simulink model "Case2_CLF_CBF_QP_Controller"  (R2026a)
settings: Solver=VariableStepAuto  StopTime=30
PreLoadFcn:
  | % Define variants
  | VSS_PATH_CTRL_PURE_PURSUIT=Simulink.Variant('VSS_PATH_CTRL_MODE==1');
  | VSS_PATH_CTRL_REAR_WHEEL=Simulink.Variant('VSS_PATH_CTRL_MODE==2');
  | % Select default variant
  | VSS_PATH_CTRL_MODE =1;
  | 
  | 
  | % Longitudinal PID
  | LongitudinalPID.Kp = 20;
  | LongitudinalPID.Ki = 0;
  | LongitudinalPID.Kd = 0;
  | LongitudinalPID.N = 100;
  | LongitudinalPID.MaxAccel = 80;
  | LongitudinalPID.SampleTime = 0.01;
  | 
  | % Steering PID
  | SteeringPID.Kp = 60;
  | SteeringPID.Ki = 0;
  | SteeringPID.Kd = 5;
  | SteeringPID.N = 10;
  | SteeringPID.MaxSpeed =  10;
  | SteeringPID.MinSpeed = -10;
  | SteeringPID.SampleTime = 0.01;
  | 
  | 
  | 
  | setSMVehicleVisuParameters;
  | 
  | % Load planner commands
  | load('PlannerCmdTests.mat');
  | % Assign one for testing:
  | plannerCmd = plannerCmdFwd;
  | % plannerCmd  = plannerCmdFwdBwd;
  | 
  | % Bus structure definition
  | load('PlannerBusStruct.mat');
  | 
  | % Rear Wheel Controller Parameters
  | RW.k_e = 0.2;    % 0.1
  | RW.k_theta = 1;   % 0.75
  | RW.SampleTime =  0.1;
  | RW.GoalRadius = 0.3;
  | 
  | % Pure pursuit parameters
  | PP.DesiredLinearVel = 5;
  | PP.MaxAngularVel  = 10;
  | PP.LookaheadDist  = 1;
  | PP.Wheelbase = 4;
  | PP.GoalRadius = 0.1;
  | PP.SampleTime = 0.1;
  | PP.LongitudinalPID.Kp = 20;
  | PP.LongitudinalPID.Ki = 0;
  | PP.LongitudinalPID.Kd = 0;
  | PP.LongitudinalPID.N = 100;
  | PP.LongitudinalPID.MaxLongAccel =  80;
  | PP.LongitudinalPID.MinLongAccel = -80;
  | 
  | % Spline ref
  | splineRef = [ 0 0 0;[plannerCmd.PathMatrix(1:plannerCmd.PathLengths(1),1:2,1),0*ones(length(plannerCmd.PathMatrix(1:plannerCmd.PathLengths(1),1,1)),1)]];
values from neighbouring files (symbols this model uses):
  m = max(2, ceil(Lseg/ds))    [Trajectory.m]    (also in plot_nmpc_result.m = NaN)
  s = [0; cumsum(hypot(diff(xs),diff(ys)))]    [Trajectory.m]    (also in plot_parking_mpc.m = evalin('base',name); plot_result.m = out.(names{k}))
  trajMatrix = [tvec, xd, yd, thd, vd, wd]    [Trajectory.m]    (also in plot_parking_mpc.m = evalin('base','trajMatrix'); plot_result.m = evalin('base','trajMatrix'))
undefined symbols (not defined in the file or in its folder): DiscIntNeverNeededParam, smvv, X, Y, Z
libraries: sm_lib x527, sm_vehicle_slalom_lib x48, fl_lib x40, fl_ps_legacy_lib x28, nesl_utility x13
(part 1 of 15)
settings Model: Creator=csantacr  LastModifiedBy=Sea
settings DataIOCC: LoggingToFile=on
settings SimscapeCC: SimscapeNormalizeSystem=off  SimscapeNominalValues="[{\"value\":\"1\",\"unit\":\"A\"},{\"value\":\"1\",\"unit\":\"bar\"},{\"value\":\"1\",\"unit\":\"cm^2\"},{\"value\":\"1\",\"unit\":\"cm^3/s\"},{\"value\":\"1\",\"unit\":\"kJ/kg\"},{\"value\":\"1\",\"unit\":\"kW\"},{\"value\":\"1\",\"unit\":\"l\"},{\"value\":\"1\",\"unit\":\"N\"},{\"value\":\"1\",\"unit\":\"N*m\"},{\"value\":\"1\",\"unit\":\"V\"}]"  SimscapeLogType=none  SimscapeLogDataHistory=5000.0
settings ExplorerConfigSet: InternalSimMechanicsExplorerSettings="<ExplorerConfiguration><canonicalview>default</canonicalview><AnimationSetting><BasePlaybackSpeed>1.0</BasePlaybackSpeed><PlaybackSpeedFactor>1.0</PlaybackSpeedFactor></AnimationSetting><TilePanel><TileInfo><Tiles Columns=\"1\" Count=\"2\" Rows=\"2\"><Column Weight=\"1\"/><Row Weight=\"0.4993\"/><Row Weight=\"0.5007\"/><Tile Height=\"1\" Width=\"1\" X=\"0\" Y=\"0\"/><Tile Height=\"1\" Width=\"1\" X=\"0\" Y=\"1\"/></Tiles></TileInfo><SceneInfo><SceneViewer><BGColor><R>0.60000002384185791</R><G>0.60000002384185791</G><B>0.60000002384185791</B></BGColor><Camera><DoPerspective>off</DoPerspective><Position><X>122.753178902162432</X><Y>-60.2531801004264622</Y><Z>85.3731797239170476</Z></Position><Center><X>37.3783324220490201</X><Y>25.1216663796874506</Y><Z>-0.00166675619682621345</Z></Center><Up><X>-0.408248290463863073</X><Y>0.408248290463863073</Y><Z>0.816496580927726145</Z></Up><ViewLimDist>1</ViewLimDist><YLim>29.4844991357607569</YLim><XLim>45.8841613769531307</XLim></Camera></SceneViewer><SceneViewer><BGColor><R>0.60000002384185791</R><G>0.60000002384185791</G><B>0.60000002384185791</B></BGColor><Camera><DoPerspective>on</DoPerspective><Position><X>8</X><Y>0</Y><Z>2</Z></Position><Center><X>0</X><Y>0.25</Y><Z>1.30299999999999994</Z></Center><Up><X>-2.22044604925031308e-16</X><Y>0</Y><Z>1</Z></Up><ViewLimDist>1</ViewLimDist><YLim>0.466307658154998583</YLim><XLim>0.72353341648828684</XLim></Camera></SceneViewer></SceneInfo></TilePanel><MechEditorPanel><Cameras><Camera><Id>Camera1</Id><Value><Name>DriverCamera</Name><NativeCamera><PositionTrackingFeature>Robot_Bicycle_Model.Visualizer.SM_Car_Visu.Vehicle1.Drivers_View_Cam.F</PositionTrackingFeature><CenterTrackingFeature>Robot_Bicycle_Model.Visualizer.SM_Car_Visu.Vehicle1.Drivers_View_Cam.F</CenterTrackingFeature><UpVectorTrackingFeature>Robot_Bicycle_Model.Visualizer.SM_Car_Visu.Vehicle1.Drivers_View_Cam.F</UpVectorTrackingFeature><CenterTrackingOrigin>off</CenterTrackingOrigin><CenterTrackingDirection>+X</CenterTrackingDirection><UpVectorTrackingDirection>+Z</UpVectorTrackingDirection></NativeCamera></Value></Camera><Camera><Id>Camera2</Id><Value><Name>FollowerX</Name><NativeCamera><PositionTrackingFeature>Robot_Bicycle_Model.Visualizer.SM_Car_Visu.Cameras_Frames.Front_View_Cam.F</PositionTrackingFeature><CenterTrackingFeature>Robot_Bicycle_Model.Visualizer.SM_Car_Visu.Vehicle1.Drivers_View_Cam.F</CenterTrackingFeature><UpVectorTrackingFeature>Robot_Bicycle_Model.Visualizer.SM_Car_Visu.Cameras_Frames.Front_View_Cam.F</UpVectorTrackingFeature><CenterTrackingOrigin>on</CenterTrackingOrigin><UpVectorTrackingDirection>-X</UpVectorTrackingDirection></NativeCamera></Value></Camera></Cameras><GfxPanelCameraMap><MapElement CameraMLId=\"Camera2\" GfxPanelIndex=\"1\"/></GfxPanelCameraMap><VideoCreator><PlaybackSpeedRatio>1.0</PlaybackSpeedRatio><FrameRate>30</FrameRate><VideoFormat>Motion JPEG AVI</VideoFormat><FrameSize>auto</FrameSize></VideoCreator></MechEditorPanel></ExplorerConfiguration>"

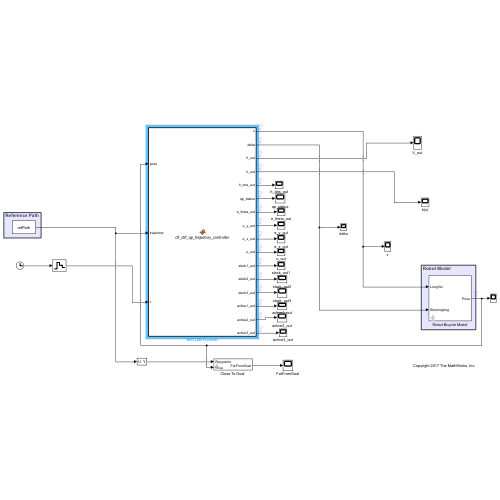
[thumbnail: Simulink's stored preview of the top-level diagram]
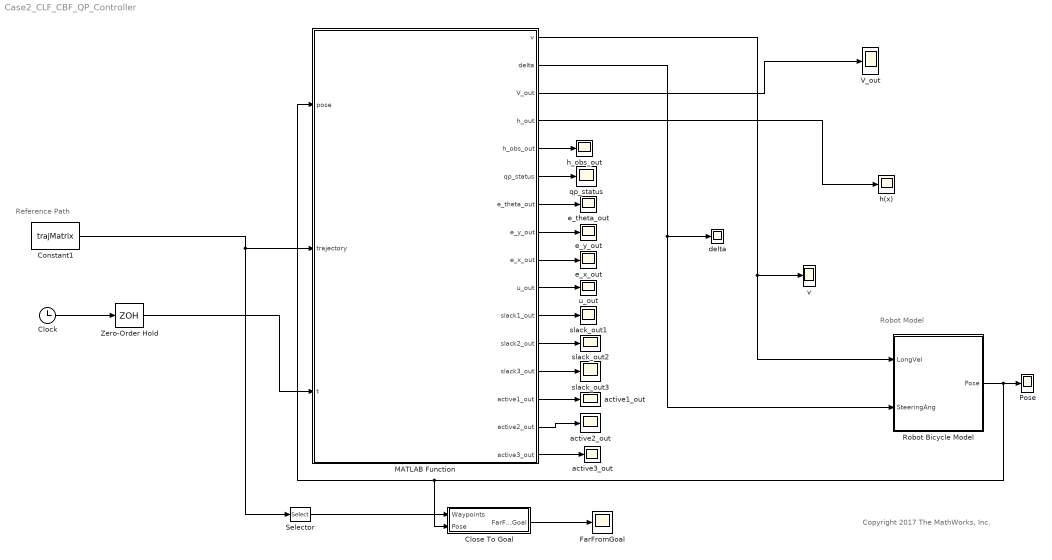
== system Case2_CLF_CBF_QP_Controller ==
  note: Copyright 2017 The MathWorks, Inc.
  note: Robot Model
  note: Reference Path
  Clock : Clock
  "Close To Goal " : Subsystem  mask{goalRadius=PP.GoalRadius}
      mask prompts: goalRadius "Goal Radius"
      mask DialogControl DescGroupVar Prompt: Close To Goal
      mask DialogControl DescTextVar Prompt: Check if close to goal
  Constant1 : Constant  Value=trajMatrix  VectorParams1D=off
      mask Display: disp('refPath');
  FarFromGoal : Scope
      settings: ActiveDisplayYMinimum=0.9  ActiveDisplayYMaximum=1.1  DataLoggingVariableName=ScopeData10
  MATLAB Function : MATLAB Function  TreatAsAtomicUnit=on  SystemSampleTime=0.01
  Pose : Scope
      settings: ActiveDisplayYMinimum=-6.9296030916089348  ActiveDisplayYMaximum=59.429979148987471  DataLoggingVariableName=pose_log
  Robot Bicycle Model : Subsystem  mask{wheelBase=3, maxLinearVelocity=80, sampleTime=5e-3, maxSteeringAng=60*pi/180, state_0=[0 16.36 0]}
      mask prompts: wheelBase "Wheel Base [m]"; maxLinearVelocity "Maximum Linear Velocity [m/s]"; sampleTime "Sample Time [s]"; maxSteeringAng "Max Steering Ang [rad]"; state_0 "Initial Condition [x,y,theta]"
  Selector : Selector  NumberOfDimensions=2  InputPortWidth=3  IndexOptions=Select all,Index vector (dialog)  Indices=[1 3],[2 3]  OutputSizes=1,1
  V_out : Scope
      settings: ActiveDisplayYMinimum=-0.032645596625243516  ActiveDisplayYMaximum=0.2938103696271917  DataLoggingVariableName=Vout_log
  Zero-Order Hold : ZeroOrderHold  SampleTime=0.01
  active1_out : Scope
      settings: ActiveDisplayYMinimum=-0.12499999999999997  ActiveDisplayYMaximum=1.125  DataLoggingVariableName=active1_log
  active2_out : Scope
      settings: DataLoggingVariableName=active2_log
  active3_out : Scope
      settings: DataLoggingVariableName=active3_log
  delta : Scope
      settings: ActiveDisplayYMinimum=-1.0989870972877505  ActiveDisplayYMaximum=1.1230265089850515  DataLoggingVariableName=delta_log
  e_theta_out : Scope
      settings: ActiveDisplayYMinimum=-1  ActiveDisplayYMaximum=1  DataLoggingVariableName=eth_log
  e_x_out : Scope
      settings: ActiveDisplayYMinimum=-3.0596180061562785  ActiveDisplayYMaximum=3.0448929725725327  DataLoggingVariableName=ex_log
  e_y_out : Scope
      settings: ActiveDisplayYMinimum=-1  ActiveDisplayYMaximum=1  DataLoggingVariableName=ey_log
  h(x) : Scope
      settings: ActiveDisplayYMinimum=-0.22434897213807364  ActiveDisplayYMaximum=1.9287865372378259  DataLoggingVariableName=h_log
  h_obs_out : Scope
      settings: ActiveDisplayYMinimum=-212.92680425947211  ActiveDisplayYMaximum=1992.0909004482746  DataLoggingVariableName=hobs_log
  qp_status : Scope
      settings: ActiveDisplayYMinimum=-1  ActiveDisplayYMaximum=1  DataLoggingVariableName=qp_log
  slack_out1 : Scope
      settings: DataLoggingVariableName=slack1_log
  slack_out2 : Scope
      settings: DataLoggingVariableName=slack2_log
  slack_out3 : Scope
      settings: DataLoggingVariableName=slack3_log
  u_out : Scope
      settings: ActiveDisplayYMinimum=-1  ActiveDisplayYMaximum=1  DataLoggingVariableName=ScopeData9
  v : Scope
      settings: ActiveDisplayYMinimum=-2.1757249365262057  ActiveDisplayYMaximum=4.581524428735853  DataLoggingVariableName=v_log
  wires:
  MATLAB Function/3(V_out) -> V_out/1
  Clock/1 -> Zero-Order Hold/1
  Zero-Order Hold/1 -> MATLAB Function/3(t)
  MATLAB Function/5(h_obs_out) -> h_obs_out/1
  Constant1/1 -> Selector/1, MATLAB Function/2(trajectory)
  Robot Bicycle Model/1(Pose) -> "Close To Goal "/2(Pose), MATLAB Function/1(pose), Pose/1
  MATLAB Function/4(h_out) -> h(x)/1
  Selector/1 -> "Close To Goal "/1(Waypoints)
  "Close To Goal "/1(FarFromGoal) -> FarFromGoal/1
  MATLAB Function/1(v) -> Robot Bicycle Model/1(LongVel), v/1
  MATLAB Function/2(delta) -> Robot Bicycle Model/2(SteeringAng), delta/1
  MATLAB Function/6(qp_status) -> qp_status/1
  MATLAB Function/7(e_theta_out) -> e_theta_out/1
  MATLAB Function/8(e_y_out) -> e_y_out/1
  MATLAB Function/9(e_x_out) -> e_x_out/1
  MATLAB Function/10(u_out) -> u_out/1
  MATLAB Function/11(slack1_out) -> slack_out1/1
  MATLAB Function/12(slack2_out) -> slack_out2/1
  MATLAB Function/13(slack3_out) -> slack_out3/1
  MATLAB Function/14(active1_out) -> active1_out/1
  MATLAB Function/15(active2_out) -> active2_out/1
  MATLAB Function/16(active3_out) -> active3_out/1

== system Case2_CLF_CBF_QP_Controller/Close To Goal  ==
  Waypoints : Inport
  Pose : Inport  Port=2
  " Extract Goal" : MATLAB Function  TreatAsAtomicUnit=on
  Data Type Conversion : DataTypeConversion  OutDataTypeStr=double  SaturateOnIntegerOverflow=off  RndMeth=Floor
  Dot Product : DotProduct  OutDataTypeStr=Inherit: Inherit via internal rule
  GoalRadius : Constant  Value=goalRadius
  Logical Operator : Logic  Operator=NOT  AllPortsSameDT=off  OutDataTypeStr=boolean
  Relational Operator : RelationalOperator  Operator=<=  OutDataTypeStr=boolean  RndMeth=Simplest  InputSameDT=off
  Selector : Selector  InputPortWidth=3  IndexOptions=Index vector (dialog)  Indices=[1 2]  OutputSizes=1
  Sqrt : Sqrt
  Subtract : Sum  Inputs=+-
  FarFromGoal : Outport  VectorParamsAs1DForOutWhenUnconnected=off
  wires:
  GoalRadius/1 -> Relational Operator/2
  Sqrt/1 -> Relational Operator/1
  Pose/1 -> Selector/1
  " Extract Goal"/1(Goal) -> Subtract/2
  Selector/1 -> Subtract/1
  Dot Product/1 -> Sqrt/1
  Relational Operator/1 -> Logical Operator/1
  Subtract/1 -> Dot Product/1, Dot Product/2
  Waypoints/1 -> " Extract Goal"/1(Waypoints)
  Logical Operator/1 -> Data Type Conversion/1
  Data Type Conversion/1 -> FarFromGoal/1

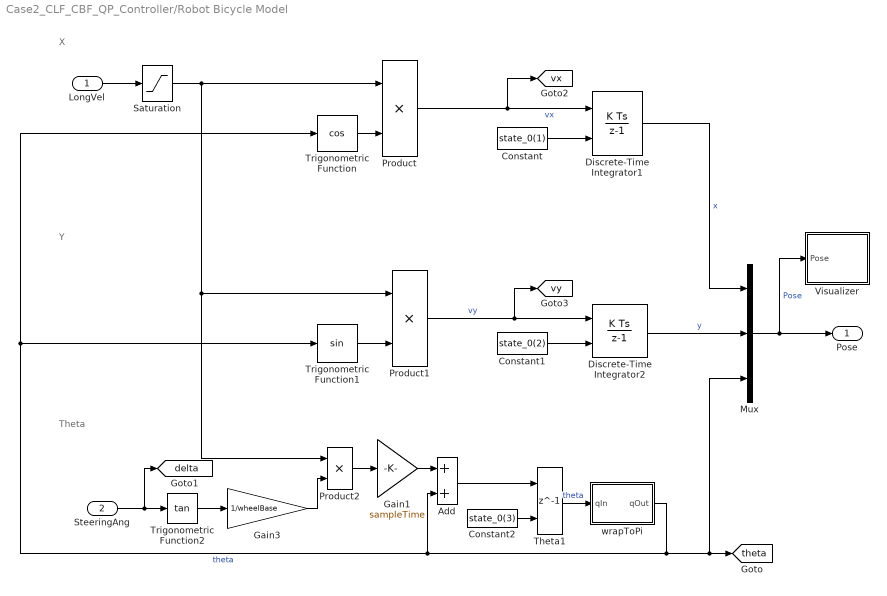
== system Case2_CLF_CBF_QP_Controller/Robot Bicycle Model ==
  note: X
  note: Y
  note: Theta
  LongVel : Inport
  SteeringAng : Inport  Port=2  SampleTime=sampleTime
  Add : Sum
  Constant : Constant  Value=state_0(1)
  Constant1 : Constant  Value=state_0(2)
  Constant2 : Constant  Value=state_0(3)
  Discrete-Time Integrator1 : DiscreteIntegrator  InitialConditionSource=external  SampleTime=-1  ICPrevOutput=DiscIntNeverNeededParam  ICPrevScaledInput=DiscIntNeverNeededParam
  Discrete-Time Integrator2 : DiscreteIntegrator  InitialConditionSource=external  SampleTime=-1  ICPrevOutput=DiscIntNeverNeededParam  ICPrevScaledInput=DiscIntNeverNeededParam
  Gain1 : Gain  Gain=sampleTime
  Gain3 : Gain  Gain=1/wheelBase
  Mux : Mux  Inputs=3
  Product : Product
  Product1 : Product
  Product2 : Product
  Saturation : Saturate  UpperLimit=maxLinearVelocity  LowerLimit=-maxLinearVelocity
  Theta1 : Delay  DelayLength=1  InitialConditionSource=Input port
      settings: InputPortMap=u0,p4
  Trigonometric Function : Trigonometry  Operator=cos
  Trigonometric Function1 : Trigonometry
  Trigonometric Function2 : Trigonometry  Operator=tan
  Visualizer : Subsystem
  wrapToPi : MATLAB Function  TreatAsAtomicUnit=on
      settings: CopyFcn=set_param(gcbh,'LinkStatus','none');
  Pose : Outport  VectorParamsAs1DForOutWhenUnconnected=off
  tag scope: delta=global, theta=global, vx=global, vy=global
  wires:
  wrapToPi/1(qOut) -> Trigonometric Function/1, Trigonometric Function1/1, Add/2, Mux/3, [theta]  "theta"
  Saturation/1 -> Product2/1, Product1/1, Product/1
  Mux/1 -> Pose/1, Visualizer/1(Pose)  "Pose"
  Theta1/1 -> wrapToPi/1(qIn)  "theta"
  Gain1/1 -> Add/1
  Add/1 -> Theta1/1
  Trigonometric Function/1 -> Product/2
  Product/1 -> [vx], Discrete-Time Integrator1/1  "vx"
  Trigonometric Function1/1 -> Product1/2
  Product1/1 -> [vy], Discrete-Time Integrator2/1  "vy"
  Product2/1 -> Gain1/1
  Constant2/1 -> Theta1/2
  Trigonometric Function2/1 -> Gain3/1
  Gain3/1 -> Product2/2
  Discrete-Time Integrator1/1 -> Mux/1  "x"
  Discrete-Time Integrator2/1 -> Mux/2  "y"
  Constant/1 -> Discrete-Time Integrator1/2
  Constant1/1 -> Discrete-Time Integrator2/2
  SteeringAng/1 -> [delta], Trigonometric Function2/1
  LongVel/1 -> Saturation/1

== system Case2_CLF_CBF_QP_Controller/Robot Bicycle Model/Visualizer ==
  Pose : Inport
  Demux : Demux  Outputs=3
  Demux1 : Demux  Outputs=2
  Earth_To_Body : Subsystem
  Extract_Vel_Steer : Subsystem
  Mux1 : Mux  Inputs=2
  Mux3 : Mux  Inputs=9
  SM_Car_Visu : Subsystem
  Terminator : Terminator
  wires:
  Demux/1 -> Mux3/1
  Demux/2 -> Mux3/2
  [theta] -> Mux3/3
  Pose/1 -> SM_Car_Visu/1(Pose_Rear), Demux/1
  Mux3/1 -> Extract_Vel_Steer/1(State)
  [vy] -> Mux1/2
  [vy] -> Mux3/5
  [vx] -> Mux3/4
  [delta] -> Mux3/7
  [vx] -> Mux1/1
  [thetaDot] -> Mux3/6
  Mux1/1 -> Earth_To_Body/1(w_v)
  [theta] -> Earth_To_Body/2(theta)
  Earth_To_Body/1(f_v) -> Demux1/1
  Demux1/1 -> Mux3/8
  Demux1/2 -> Mux3/9
  Extract_Vel_Steer/1(Long_Vel) -> SM_Car_Visu/2(Long_Vel)
  Extract_Vel_Steer/2(Steering_Ang) -> SM_Car_Visu/3(Steering_Angle)
  Demux/3 -> Terminator/1

== system Case2_CLF_CBF_QP_Controller/Robot Bicycle Model/Visualizer/Earth_To_Body ==
  w_v : Inport
  theta : Inport  Port=2
  Add : Sum
  Add1 : Sum
  Demux : Demux  Outputs=2
  Gain : Gain  Gain=-1
  Mux : Mux  Inputs=2
  Product{,1..3} (4 alike) : Product
  Trigonometric Function : Trigonometry
  Trigonometric Function1 : Trigonometry  Operator=cos
  f_v : Outport  VectorParamsAs1DForOutWhenUnconnected=off
  wires:
  Add1/1 -> Mux/2
  Product3/1 -> Add1/2
  Product2/1 -> Gain/1
  Trigonometric Function/1 -> Product1/1, Product2/2
  Add/1 -> Mux/1
  Mux/1 -> f_v/1
  Demux/2 -> Product3/2, Product1/2
  Product1/1 -> Add/2
  Product/1 -> Add/1
  Demux/1 -> Product2/1, Product/1
  w_v/1 -> Demux/1
  Trigonometric Function1/1 -> Product/2, Product3/1
  theta/1 -> Trigonometric Function/1, Trigonometric Function1/1
  Gain/1 -> Add1/1

== system Case2_CLF_CBF_QP_Controller/Robot Bicycle Model/Visualizer/Extract_Vel_Steer ==
  State : Inport
  Demux : Demux  Outputs=9
  Terminator{,1..6} (7 alike) : Terminator
  Long_Vel : Outport  VectorParamsAs1DForOutWhenUnconnected=off
  Steering_Ang : Outport  Port=2  VectorParamsAs1DForOutWhenUnconnected=off
  wires:
  State/1 -> Demux/1
  Demux/1 -> Terminator/1
  Demux/2 -> Terminator1/1
  Demux/3 -> Terminator2/1
  Demux/9 -> Terminator3/1
  Demux/4 -> Terminator4/1
  Demux/5 -> Terminator5/1
  Demux/6 -> Terminator6/1
  Demux/7 -> Steering_Ang/1
  Demux/8 -> Long_Vel/1

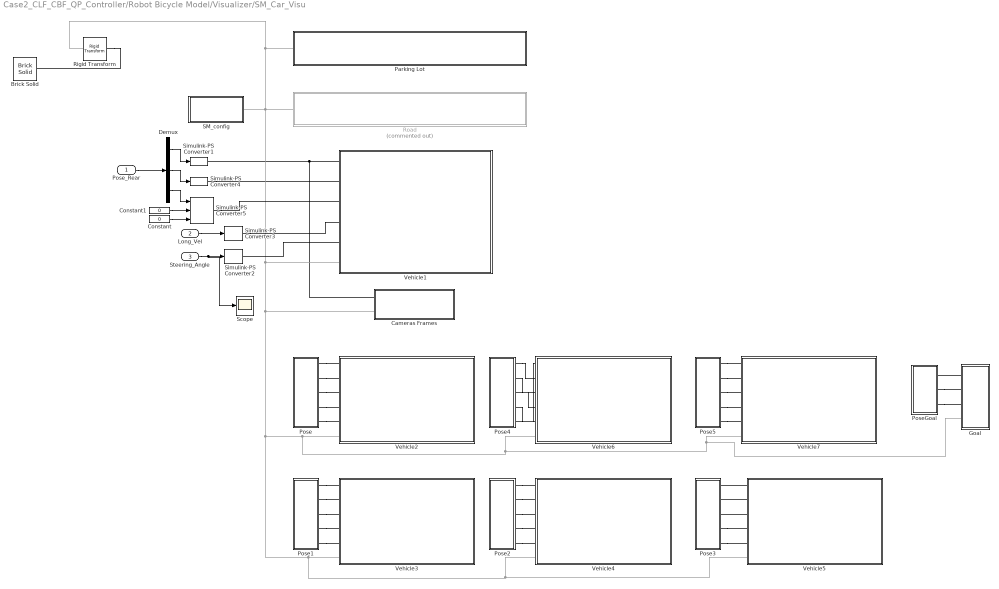
== system Case2_CLF_CBF_QP_Controller/Robot Bicycle Model/Visualizer/SM_Car_Visu ==
  Pose_Rear : Inport
  Long_Vel : Inport  Port=2
  Steering_Angle : Inport  Port=3
  Brick Solid : sm_lib/Body Elements/Brick Solid  BrickDimensions=[1 1 1]  BrickDimensionsUnits=m  ExportEntireGeometry=off  InertiaType=CalculateFromGeometry  BasedOnType=Density  Density=1000  DensityUnits=kg/m^3  Mass=1  MassUnits=kg  CenterOfMass=[0 0 0]  CenterOfMassUnits=m  MomentsOfInertia=[1 1 1]  MomentsOfInertiaUnits=kg*m^2  ProductsOfInertia=[0 0 0]  ProductsOfInertiaUnits=kg*m^2  GraphicType=FromGeometry  MarkerShape=Sphere  MarkerSize=10  GraphicVisPropType=SimpleVisualProperties  GraphicDiffuseColor=[0.3333 0.6667 0]  GraphicOpacity=1  GraphicSpecularColor=[0.5 0.5 0.5 1.0]  GraphicAmbientColor=[0.15 0.15 0.15 1.0]  GraphicEmissiveColor=[0.0 0.0 0.0 1.0]  GraphicShininess=75  DoExposeReferenceFrame=on  SerializedFrames=<Frames/>
  Cameras Frames : Subsystem
  Constant : Constant  Value=0
  Constant1 : Constant  Value=0
  Demux : Demux  Outputs=3
  Goal : Subsystem
  Parking Lot : Subsystem
  Pose : Subsystem
  Pose1 : Subsystem
  Pose2 : Subsystem
  Pose3 : Subsystem
  Pose4 : Subsystem
  Pose5 : Subsystem
  PoseGoal : Subsystem
  Rigid Transform : sm_lib/Frames and Transforms/Rigid Transform  RotationMethod=None  FollAlignAxisA=+X  BaseAlignAxisA=+Y  FollAlignAxisB=+Y  BaseAlignAxisB=+Z  RotationStandardAxis=+Z  RotationAngle=0  RotationAngleUnits=deg  RotationArbitraryAxis=[0 0 1]  RotationSequenceAxes=FollowerAxes  RotationSequence=XYX  RotationSequenceAngles=[0 0 0]  RotationSequenceAnglesUnits=deg  RotationMatrix=[1 0 0;0 1 0;0 0 1]  Quaternion=[1 0 0 0]  TranslationMethod=Cartesian  TranslationCartesianOffset=[0 17 0]  TranslationCartesianOffsetUnits=m  TranslationStandardAxis=+Z  TranslationStandardOffset=0  TranslationStandardOffsetUnits=m  TranslationROffset=0  TranslationROffsetUnits=m  TranslationThetaOffset=0  TranslationThetaOffsetUnits=deg  TranslationZOffset=0  TranslationZOffsetUnits=m
  Road : Subsystem  Commented=on
      mask Display: image(imread(fullfile(matlabroot,'toolbox','physmod','sm','smdemos','vehicle_slalom','images','sm_vehicle_slalom_road.png')));
  SM_config : Subsystem
  Scope : Scope
      settings: ActiveDisplayYMinimum=-1.10804  ActiveDisplayYMaximum=1.68533
  Simulink-PS Converter{1..4} (4 alike) : nesl_utility/Simulink-PS Converter  PhysicalDomain=network_engine_domain  SubClassName=ps_input  LeftPortType=input  RightPortType=output  PseudoPeriodic=off  Frequencies=[]  NoiseDistribution=none  NoiseParameters=[]  Unit=1  AffineConversion=off  FilteringAndDerivatives=filter  SimscapeFilterOrder=2  InputFilterTimeConstant=smvv.filter.t_c  UdotUserProvided=2
  Simulink-PS Converter5 : nesl_utility/Simulink-PS Converter  PhysicalDomain=network_engine_domain  SubClassName=ps_input  LeftPortType=input  RightPortType=output  PseudoPeriodic=off  Frequencies=[]  NoiseDistribution=none  NoiseParameters=[]  Unit=rad  AffineConversion=off  FilteringAndDerivatives=provide  SimscapeFilterOrder=2  InputFilterTimeConstant=smvv.filter.t_c  UdotUserProvided=2
  Vehicle1 : Subsystem
      mask Display: image(imread(fullfile(matlabroot,'toolbox','physmod','sm','smdemos','vehicle_slalom','images','sm_vehicle_slalom_vehicle.png')));
  Vehicle2 : Subsystem
      mask Display: image(imread(fullfile(matlabroot,'toolbox','physmod','sm','smdemos','vehicle_slalom','images','sm_vehicle_slalom_vehicle.png')));
  Vehicle3 : Subsystem
      mask Display: image(imread(fullfile(matlabroot,'toolbox','physmod','sm','smdemos','vehicle_slalom','images','sm_vehicle_slalom_vehicle.png')));
  Vehicle4 : Subsystem
      mask Display: image(imread(fullfile(matlabroot,'toolbox','physmod','sm','smdemos','vehicle_slalom','images','sm_vehicle_slalom_vehicle.png')));
  Vehicle5 : Subsystem
      mask Display: image(imread(fullfile(matlabroot,'toolbox','physmod','sm','smdemos','vehicle_slalom','images','sm_vehicle_slalom_vehicle.png')));
  Vehicle6 : Subsystem
      mask Display: image(imread(fullfile(matlabroot,'toolbox','physmod','sm','smdemos','vehicle_slalom','images','sm_vehicle_slalom_vehicle.png')));
  Vehicle7 : Subsystem
      mask Display: image(imread(fullfile(matlabroot,'toolbox','physmod','sm','smdemos','vehicle_slalom','images','sm_vehicle_slalom_vehicle.png')));
  wires:
  Demux/2 -> Simulink-PS Converter4/1
  Pose_Rear/1 -> Demux/1
  Demux/3 -> Simulink-PS Converter5/1
  Demux/1 -> Simulink-PS Converter1/1
  Steering_Angle/1 -> Scope/1, Simulink-PS Converter2/1
  Long_Vel/1 -> Simulink-PS Converter3/1
  Constant/1 -> Simulink-PS Converter5/3
  Constant1/1 -> Simulink-PS Converter5/2
  connections:
  Simulink-PS Converter4/RConn1 -- Vehicle1/LConn2
  Cameras Frames/LConn1 -- Vehicle1/LConn1 -- Simulink-PS Converter1/RConn1
  Road/LConn1 -- Parking Lot/LConn1 -- Rigid Transform/LConn1 -- SM_config/RConn1 -- Vehicle1/LConn6 -- Goal/LConn4 -- Vehicle7/LConn6 -- Vehicle6/LConn6 -- Vehicle2/LConn6 -- Vehicle5/LConn6 -- Vehicle4/LConn6 -- Vehicle3/LConn6 -- Cameras Frames/LConn2
  Vehicle1/LConn5 -- Simulink-PS Converter2/RConn1
  Simulink-PS Converter5/RConn1 -- Vehicle1/LConn3
  Simulink-PS Converter3/RConn1 -- Vehicle1/LConn4
  Pose/RConn1 -- Vehicle2/LConn1
  Pose/RConn2 -- Vehicle2/LConn2
  Pose/RConn3 -- Vehicle2/LConn3
  Pose/RConn4 -- Vehicle2/LConn4
  Pose/RConn5 -- Vehicle2/LConn5
  Pose1/RConn1 -- Vehicle3/LConn1
  Pose1/RConn2 -- Vehicle3/LConn2
  Pose1/RConn3 -- Vehicle3/LConn3
  Pose1/RConn4 -- Vehicle3/LConn4
  Pose1/RConn5 -- Vehicle3/LConn5
  Pose2/RConn1 -- Vehicle4/LConn1
  Pose2/RConn2 -- Vehicle4/LConn2
  Pose2/RConn3 -- Vehicle4/LConn3
  Pose2/RConn4 -- Vehicle4/LConn4
  Pose2/RConn5 -- Vehicle4/LConn5
  Vehicle5/LConn3 -- Pose3/RConn3
  Vehicle5/LConn2 -- Pose3/RConn2
  Vehicle5/LConn1 -- Pose3/RConn1
  Pose3/RConn4 -- Vehicle5/LConn4
  Pose3/RConn5 -- Vehicle5/LConn5
  Pose4/RConn3 -- Vehicle6/LConn4
  Pose4/RConn2 -- Vehicle6/LConn3
  Pose4/RConn1 -- Vehicle6/LConn2
  Pose4/RConn5 -- Vehicle6/LConn1
  Pose4/RConn4 -- Vehicle6/LConn5
  Pose5/RConn2 -- Vehicle7/LConn2
  Pose5/RConn1 -- Vehicle7/LConn1
  Pose5/RConn3 -- Vehicle7/LConn3
  Pose5/RConn4 -- Vehicle7/LConn4
  Pose5/RConn5 -- Vehicle7/LConn5
  Goal/LConn1 -- PoseGoal/RConn1
  PoseGoal/RConn2 -- Goal/LConn2
  PoseGoal/RConn3 -- Goal/LConn3
  Rigid Transform/RConn1 -- Brick Solid/RConn1

== system Case2_CLF_CBF_QP_Controller/Robot Bicycle Model/Visualizer/SM_Car_Visu/Cameras Frames ==
  Alignment xForm : sm_lib/Frames and Transforms/Rigid Transform  RotationMethod=AlignedAxes  FollAlignAxisA=+Z  BaseAlignAxisA=+X  FollAlignAxisB=+Y  BaseAlignAxisB=+Y  RotationStandardAxis=+Z  RotationAngle=0.0  RotationAngleUnits=deg  RotationArbitraryAxis=[0 0 1]  RotationSequenceAxes=FollowerAxes  RotationSequence=XYX  RotationSequenceAngles=[0 0 0]  RotationSequenceAnglesUnits=deg  RotationMatrix=[1 0 0; 0 1 0; 0 0 1]  Quaternion=[1 0 0 0]  TranslationMethod=None  TranslationCartesianOffset=[0 0 0]  TranslationCartesianOffsetUnits=m  TranslationStandardAxis=+Z  TranslationStandardOffset=0  TranslationStandardOffsetUnits=m  TranslationROffset=0  TranslationROffsetUnits=m  TranslationThetaOffset=0  TranslationThetaOffsetUnits=deg  TranslationZOffset=0  TranslationZOffsetUnits=m
  Front View xForm : sm_lib/Frames and Transforms/Rigid Transform  RotationMethod=None  FollAlignAxisA=+X  BaseAlignAxisA=+Y  FollAlignAxisB=+Y  BaseAlignAxisB=+Z  RotationStandardAxis=+Z  RotationAngle=0.0  RotationAngleUnits=deg  RotationArbitraryAxis=[0 0 1]  RotationSequenceAxes=FollowerAxes  RotationSequence=XYX  RotationSequenceAngles=[0 0 0]  RotationSequenceAnglesUnits=deg  RotationMatrix=[1 0 0; 0 1 0; 0 0 1]  Quaternion=[1 0 0 0]  TranslationMethod=Cartesian  TranslationCartesianOffset=smvv.cameras.frontView_offset  TranslationCartesianOffsetUnits=m  TranslationStandardAxis=+Z  TranslationStandardOffset=0  TranslationStandardOffsetUnits=m  TranslationROffset=0  TranslationROffsetUnits=m  TranslationThetaOffset=0  TranslationThetaOffsetUnits=deg  TranslationZOffset=0  TranslationZOffsetUnits=m
  Front View Cam : Subsystem
  Prismatic Joint : sm_lib/Joints/Prismatic Joint  JointMode=Normal  CompositeWrenchDir=FollowerOnBase  CompositeWrenchFrame=BaseFrame  SenseConstraintForce=off  SenseConstraintTorque=off  SenseTotalForce=off  SenseTotalTorque=off  PositionTargetSpecify=on  PositionTargetPriority=High  PositionTargetValue=smvv.vehicle.posX_0  PositionTargetValueUnits=m  VelocityTargetSpecify=off  VelocityTargetPriority=High  VelocityTargetValue=0  VelocityTargetValueUnits=m/s  EquilibriumPosition=0  EquilibriumPositionUnits=m  SpringStiffness=0  SpringStiffnessUnits=N/m  DampingCoefficient=0  DampingCoefficientUnits=N/(m/s)  LowerLimitSpecify=off  LowerLimitBound=-1  LowerLimitBoundUnits=m  LowerLimitStiffness=1e6  LowerLimitStiffnessUnits=N/m  LowerLimitDamping=1e3  LowerLimitDampingUnits=N/(m/s)  LowerLimitTransitionRegionWidth=1e-4  LowerLimitTransitionRegionWidthUnits=m  UpperLimitSpecify=off  UpperLimitBound=1  UpperLimitBoundUnits=m  UpperLimitStiffness=1e6  UpperLimitStiffnessUnits=N/m  UpperLimitDamping=1e3  UpperLimitDampingUnits=N/(m/s)  UpperLimitTransitionRegionWidth=1e-4  UpperLimitTransitionRegionWidthUnits=m  TorqueActuationMode=ComputedTorque  MotionActuationMode=InputMotion  SensePosition=off  SenseVelocity=off  SenseAcceleration=off  SenseTorqueForce=off  SenseLowerLimitTorqueForce=off  SenseUpperLimitTorqueForce=off
  Side View xForm : sm_lib/Frames and Transforms/Rigid Transform  RotationMethod=None  FollAlignAxisA=+X  BaseAlignAxisA=+Y  FollAlignAxisB=+Y  BaseAlignAxisB=+Z  RotationStandardAxis=+Z  RotationAngle=0.0  RotationAngleUnits=deg  RotationArbitraryAxis=[0 0 1]  RotationSequenceAxes=FollowerAxes  RotationSequence=XYX  RotationSequenceAngles=[0 0 0]  RotationSequenceAnglesUnits=deg  RotationMatrix=[1 0 0; 0 1 0; 0 0 1]  Quaternion=[1 0 0 0]  TranslationMethod=Cartesian  TranslationCartesianOffset=smvv.cameras.sideView_offset  TranslationCartesianOffsetUnits=m  TranslationStandardAxis=+Z  TranslationStandardOffset=0  TranslationStandardOffsetUnits=m  TranslationROffset=0  TranslationROffsetUnits=m  TranslationThetaOffset=0  TranslationThetaOffsetUnits=deg  TranslationZOffset=0  TranslationZOffsetUnits=m
  Side View Cam : Subsystem
  Px : PMIOPort  Side=Left
  W : PMIOPort  Port=2  Side=Left
  connections:
  Prismatic Joint/LConn2 -- Px/RConn1
  Front View xForm/LConn1 -- Side View xForm/LConn1 -- Prismatic Joint/RConn1
  Prismatic Joint/LConn1 -- Alignment xForm/RConn1
  W/RConn1 -- Alignment xForm/LConn1
  Front View xForm/RConn1 -- Front View Cam/RConn1
  Side View Cam/RConn1 -- Side View xForm/RConn1

== system Case2_CLF_CBF_QP_Controller/Robot Bicycle Model/Visualizer/SM_Car_Visu/Goal ==
  Cartesian Joint : sm_lib/Joints/Cartesian Joint  JointMode=Normal  CompositeWrenchDir=FollowerOnBase  CompositeWrenchFrame=BaseFrame  SenseConstraintForce=off  SenseConstraintTorque=off  SenseTotalForce=off  SenseTotalTorque=off  PxPositionTargetSpecify=off  PxPositionTargetPriority=High  PxPositionTargetValue=0  PxPositionTargetValueUnits=m  PxVelocityTargetSpecify=off  PxVelocityTargetPriority=High  PxVelocityTargetValue=0  PxVelocityTargetValueUnits=m/s  PxEquilibriumPosition=0  PxEquilibriumPositionUnits=m  PxSpringStiffness=0  PxSpringStiffnessUnits=N/m  PxDampingCoefficient=0  PxDampingCoefficientUnits=N/(m/s)  PxLowerLimitSpecify=off  PxLowerLimitBound=-1  PxLowerLimitBoundUnits=m  PxLowerLimitStiffness=1e6  PxLowerLimitStiffnessUnits=N/m  PxLowerLimitDamping=1e3  PxLowerLimitDampingUnits=N/(m/s)  PxLowerLimitTransitionRegionWidth=1e-4  PxLowerLimitTransitionRegionWidthUnits=m  PxUpperLimitSpecify=off  PxUpperLimitBound=1  PxUpperLimitBoundUnits=m  PxUpperLimitStiffness=1e6  PxUpperLimitStiffnessUnits=N/m  PxUpperLimitDamping=1e3  PxUpperLimitDampingUnits=N/(m/s)  PxUpperLimitTransitionRegionWidth=1e-4  PxUpperLimitTransitionRegionWidthUnits=m  PxTorqueActuationMode=ComputedTorque  PxMotionActuationMode=InputMotion  PxSensePosition=off  PxSenseVelocity=off  PxSenseAcceleration=off  PxSenseTorqueForce=off  PxSenseLowerLimitTorqueForce=off  PxSenseUpperLimitTorqueForce=off  PyPositionTargetSpecify=off  PyPositionTargetPriority=High  PyPositionTargetValue=0  PyPositionTargetValueUnits=m  PyVelocityTargetSpecify=off  PyVelocityTargetPriority=High  PyVelocityTargetValue=0  PyVelocityTargetValueUnits=m/s  PyEquilibriumPosition=0  PyEquilibriumPositionUnits=m  PySpringStiffness=0  PySpringStiffnessUnits=N/m  PyDampingCoefficient=0  PyDampingCoefficientUnits=N/(m/s)  PyLowerLimitSpecify=off  PyLowerLimitBound=-1  PyLowerLimitBoundUnits=m  PyLowerLimitStiffness=1e6  PyLowerLimitStiffnessUnits=N/m  PyLowerLimitDamping=1e3  PyLowerLimitDampingUnits=N/(m/s)  PyLowerLimitTransitionRegionWidth=1e-4  PyLowerLimitTransitionRegionWidthUnits=m  PyUpperLimitSpecify=off  PyUpperLimitBound=1  PyUpperLimitBoundUnits=m  PyUpperLimitStiffness=1e6  PyUpperLimitStiffnessUnits=N/m  PyUpperLimitDamping=1e3  PyUpperLimitDampingUnits=N/(m/s)  PyUpperLimitTransitionRegionWidth=1e-4  PyUpperLimitTransitionRegionWidthUnits=m  PyTorqueActuationMode=ComputedTorque  PyMotionActuationMode=InputMotion  PySensePosition=off  PySenseVelocity=off  PySenseAcceleration=off  PySenseTorqueForce=off  PySenseLowerLimitTorqueForce=off  PySenseUpperLimitTorqueForce=off  PzPositionTargetSpecify=off  PzPositionTargetPriority=High  PzPositionTargetValue=0  PzPositionTargetValueUnits=m  PzVelocityTargetSpecify=off  PzVelocityTargetPriority=High  PzVelocityTargetValue=0  PzVelocityTargetValueUnits=m/s  PzEquilibriumPosition=0  PzEquilibriumPositionUnits=m  PzSpringStiffness=0  PzSpringStiffnessUnits=N/m  PzDampingCoefficient=0  PzDampingCoefficientUnits=N/(m/s)  PzLowerLimitSpecify=off  PzLowerLimitBound=-1  PzLowerLimitBoundUnits=m  PzLowerLimitStiffness=1e6  PzLowerLimitStiffnessUnits=N/m  PzLowerLimitDamping=1e3  PzLowerLimitDampingUnits=N/(m/s)  PzLowerLimitTransitionRegionWidth=1e-4  PzLowerLimitTransitionRegionWidthUnits=m  PzUpperLimitSpecify=off  PzUpperLimitBound=1  PzUpperLimitBoundUnits=m  PzUpperLimitStiffness=1e6  PzUpperLimitStiffnessUnits=N/m  PzUpperLimitDamping=1e3  PzUpperLimitDampingUnits=N/(m/s)  PzUpperLimitTransitionRegionWidth=1e-4  PzUpperLimitTransitionRegionWidthUnits=m  PzTorqueActuationMode=ComputedTorque  PzMotionActuationMode=InputMotion  PzSensePosition=off  PzSenseVelocity=off  PzSenseAcceleration=off  PzSenseTorqueForce=off  PzSenseLowerLimitTorqueForce=off  PzSenseUpperLimitTorqueForce=off
  Solid : sm_lib/Body Elements/Cylindrical Solid  CylinderRadius=0.5  CylinderRadiusUnits=m  CylinderLength=0.1  CylinderLengthUnits=m  ExportEntireGeometry=off  InertiaType=CalculateFromGeometry  BasedOnType=Density  Density=1000  DensityUnits=kg/m^3  Mass=1  MassUnits=kg  CenterOfMass=[0 0 0]  CenterOfMassUnits=m  MomentsOfInertia=[1 1 1]  MomentsOfInertiaUnits=kg*m^2  ProductsOfInertia=[1 1 1]  ProductsOfInertiaUnits=kg*m^2  GraphicType=FromGeometry  MarkerShape=Sphere  MarkerSize=10  GraphicVisPropType=SimpleVisualProperties  GraphicDiffuseColor=[1.0 1.0 1.0]  GraphicOpacity=1.0  GraphicSpecularColor=[0.5 0.5 0.5 1.0]  GraphicAmbientColor=[0.15 0.15 0.15 1.0]  GraphicEmissiveColor=[0.0 0.0 0.0 1.0]  GraphicShininess=75  DoExposeReferenceFrame=on  SerializedFrames=<Frames/>
  x : PMIOPort  Side=Left
  y : PMIOPort  Port=2  Side=Left
  z : PMIOPort  Port=3  Side=Left
  B : PMIOPort  Port=4  Side=Left
  connections:
  Cartesian Joint/LConn4 -- z/RConn1
  Cartesian Joint/LConn3 -- y/RConn1
  Solid/RConn1 -- Cartesian Joint/RConn1
  Cartesian Joint/LConn1 -- B/RConn1
  Cartesian Joint/LConn2 -- x/RConn1
